simulink model "CHP_Test_Model"  (Simulink 8.1)
settings: Solver=ode4  StartTime=0.0  StopTime=40  FixedStep=Ts  MaxStep=1e-3  RelTol=1e-3
model workspace (MAT data in the model file):
  op_snapshot1 : opcond.OperatingPoint (value not decoded)
PostLoadFcn:
  | Ts=100e-6; HILLTOP_init;SIM_HIL=0; UnitTest_Breaker_init
InitFcn:
  | Ts=100e-6; HILLTOP_init;SIM_HIL=0; UnitTest_Breaker_init
undefined symbols (not defined in the file): fdesignblkfcn, gcbh, Left, NG_CHP, NG_CHP_lib, ph, relay_par, type, V
libraries: simulink x28, rtio_opalrt_common x21, rtlab x7, simulink_extras x6, artemis x5, powerlib x4, rteventslib x4, cables_lib x3, breaker_lib x3, rtio_generic_modbus x3, Load_lib x2, transformer_lib x2
(part 1 of 3)
settings Model: ARTEMISmethode_block_infos=$$__separator__$$CHP_Test_Model/ARTEMIS Guide$$__separator__$$  Creator=RE25624  LastModifiedBy=ed12083  BufferReuse=off
settings SolverCC: ZeroCrossAlgorithm=Adaptive
settings DataIOCC: ExternalInput=getinputstruct(op_snapshot1)  InitialState=getstatestruct(op_snapshot1)  LimitDataPoints=off  MaxDataPoints=90060  SignalLoggingSaveFormat=Dataset  SaveOutput=off  SignalLogging=off  DSMLogging=off  SaveTime=off  OutputSaveName=result
settings OptimizationCC: BlockReduction=off  OptimizeBlockIOStorage=off  BufferReuse=off  ExpressionFolding=off  LocalBlockOutputs=off
settings DebuggingCC: MaxConsecutiveZCsMsg=warning  IgnoredZcDiagnostic=none  SolverPrmCheckMsg=none  MultiTaskRateTransMsg=warning  FcnCallInpInsideContextMsg=EnableAllAsWarning  FrameProcessingCompatibilityMsg=error  ModelReferenceExtraNoncontSigs=warning  StrictBusMsg=None
settings ModelReferenceCC: UpdateModelReferenceTargets=IfOutOfDate
settings SFSimCC: SFSimEcho=off
settings GRTTargetCC: CodeReplacementLibrary=C89/C90 (ANSI)

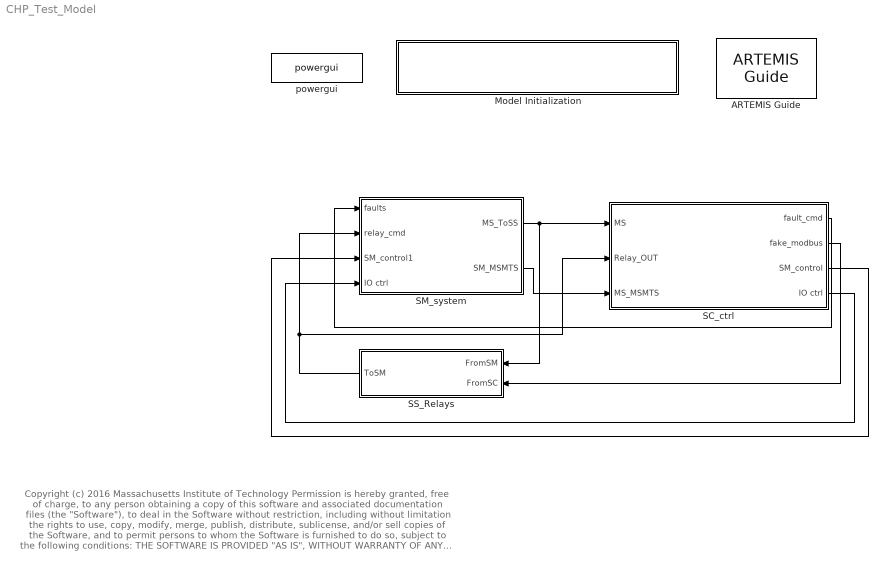
== system CHP_Test_Model ==
  note: Copyright (c) 2016 Massachusetts Institute of Technology
      | Permission is hereby granted, free of charge, to any person obtaining a copy of this software and associated documentation files (the "Software"), to deal
      | in the Software without restriction, including without limitation the rights to use, copy, modify, merge, publish, distribute, sublicense, and/or sell copies of the
      | Software, and to permit persons to whom the Software is furnished to do so, subject to the following conditions:
      |
      | THE SOFTWARE IS PROVIDED "AS IS", WITHOUT WARRANTY OF ANY KIND, EXPRESS OR IMPLIED, INCLUDING BUT NOT LIMITED TO THE
      | WARRANTIES OF MERCHANTABILITY, FITNESS FOR A PARTICULAR PURPOSE AND NONINFRINGEMENT. IN NO EVENT SHALL THE AUTHORS
      | OR COPYRIGHT HOLDERS BE LIABLE FOR ANY CLAIM, DAMAGES OR OTHER LIABILITY, WHETHER IN AN ACTION OF CONTRACT, TORT OR
      | OTHERWISE, ARISING FROM, OUT OF OR IN CONNECTION WITH THE SOFTWARE OR THE USE OR OTHER DEALINGS IN THE SOFTWARE.
  ARTEMIS Guide : artemis/ARTEMIS/ARTEMIS Guide  Tag=FTSSmethode_opal_4hx0r99  Description=5.0_z1  lock=on  Ts=Ts  opt=art5  dyna=off  nb_perm=4  RT_fullcomp=off  ssn=on  ssn_itvc=off  ssn_ivic=off  ssn_ext=off  ssn_solver=Art5 with Backward Euler nodal interface  ssn_impulse=off  ssn_quasimpulse=off  ssn_impulse_loop=2  paraExtinctionThy=off  Thy_Impulse=on  dtc=Off  dtc_opt=normal  ao=on  simtype=off  ct_mac=off  lin_mov=off  lsp=[0.001 2]  spike_skip=Disabled  dtc_extra=1  dtc_sws=normal  dtc_pied=0.5  SPSRulesBlock=SPSRules  tre=on  ctmm=off  LF=off  dpl_type=ARTEMiS DPL  rlc_type=off  custom_type=off  para=on  ssn_ImpulseLoopBlockedStateUpdate=2  ssn_mov_iter_number=5  ssn_switch_iter_number=5
  Model Initialization : Subsystem  AncestorBlock=artemis/Tools /Misc/Model Initialization  mask(Model Functions){InitFcnX=Ts=100e-6; HILLTOP_init;SIM_HIL=0; UnitTest_Breaker_init, prel=off, posl=on, inif=on, strf=off}
      mask prompts: InitFcnX "Initialisation"; prel "Preload Function"; posl "PostLoad Function"; inif "InitFcn"; strf "StartFcn"
      mask init:
      | currentBlock = gcb;
      | root = bdroot(currentBlock);
      | 
      | 
      | if ~strcmp(get_param(root,'BlockDiagramType'),'library')
      |     if prel==1
      |         set_param(root, 'PreLoadFcn', InitFcnX);
      |     else
      |         set_param(root, 'PreLoadFcn', '');
      |     end
      |     if inif==1
      |         set_param(root, 'InitFcn', InitFcnX);
      |     else
      |         set_param(root, 'InitFcn', '');
      |     end
      |     if strf==1
      |         set_param(root, 'StartFcn', InitFcnX);
      |     else
      |         set_param(root, 'StartFcn', '');
      |     end
      |     if posl==1
      |         set_param(root, 'PostLoadFcn', InitFcnX);
      |     else
      |         set_param(root, 'PostLoadFcn', '');
      |     end
      | end
      | 
      | pos = get_param(currentBlock, 'Position');
      | width = pos(3) - pos(1); height = pos(4) - pos(2);
      | txt = [ upper(root) '\n' '- InitFcn. . . . . '  get_param(root, 'InitFcn') ];
      settings: CopyFcn=set_param(gcb,'LinkStatus','inactive')
      mask Display: text(5, height*0.5, txt, 'horizontalAlignment', 'left', 'verticalAlignment', 'middle') ;
  SC_ctrl : Subsystem
  SM_system : Subsystem
  SS_Relays : Subsystem
  powergui : powerlib/powergui  Priority=2  SimulationMode=Discrete  SolverType=Tustin  SampleTime=Ts  frequency=60  SPID=off  DisableSnubberDevices=off  DisableRonSwitches=off  DisableVfSwitches=off  SwTol=0  Interpol=off  DisplayEquations=off  frequencyindice=0  Pbase=100e6  ErrMax=1e-4  Iterations=50  UnitsV=kV  UnitsW=MW  FunctionMessages=off  echomessages=off  HookPort=off  EnableUseOfTLC=off  x0status=blocks  RestoreLinks=warning  ResistiveCurrentMeasurement=off  Frange=logspace(0,3,50)  Ylog=off  Xlog=off  ShowGrid=off  save=off  variable=ZData  structure=0  ZoomFFT=on  StartTime=0.0  cycles=2  DisplayStyle=off  fundamental=60  FreqAxis=off  MaxFrequency=1000  frequencyindicesteady=1  RmsSteady=1  display=off  Ts=0  methode=off
  wires:
  SM_system/1(MS_ToSS) -> SC_ctrl/1(MS), SS_Relays/1(FromSM)
  SC_ctrl/1(fault_cmd) -> SM_system/1(faults)
  SS_Relays/1(ToSM) -> SM_system/2(relay_cmd), SC_ctrl/2(Relay_OUT)
  SC_ctrl/2(fake_modbus) -> SS_Relays/2(FromSC)
  SM_system/2(SM_MSMTS) -> SC_ctrl/3(MS_MSMTS)
  SC_ctrl/4(IO ctrl) -> SM_system/4(IO ctrl)
  SC_ctrl/3(SM_control) -> SM_system/3(SM_control1)

== system CHP_Test_Model/Model Initialization ==

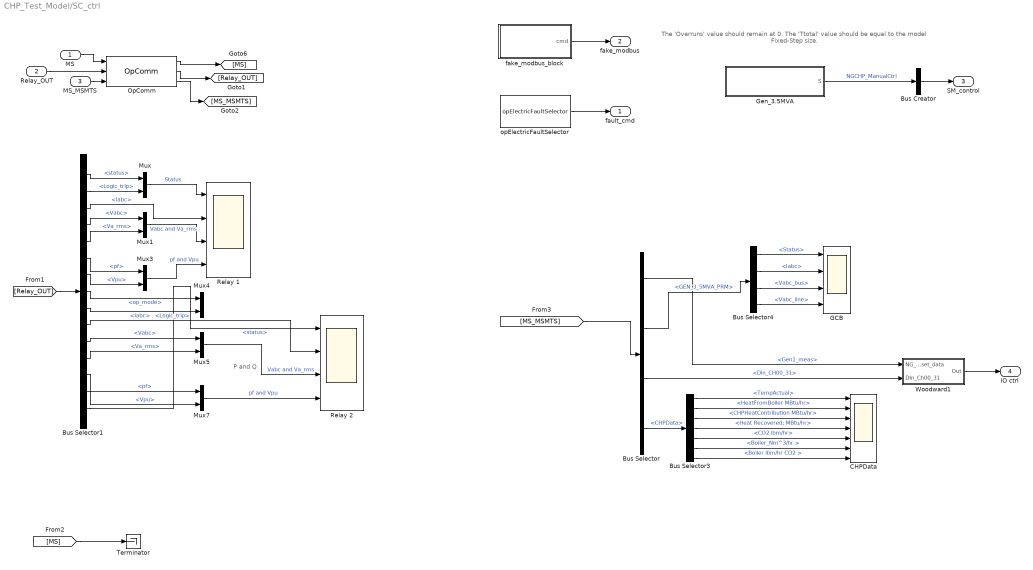
== system CHP_Test_Model/SC_ctrl ==
  note: P and Q
  note: The 'Overruns' value should remain at 0.
      | The 'Ttotal' value should be equal to the
      | model Fixed-Step size.
  MS : Inport
  Relay_OUT : Inport  Port=2
  MS_MSMTS : Inport  Port=3
  Bus Creator : BusCreator  Inputs=1
  Bus Selector : BusSelector  OutputSignals=Gen1_meas,GEN_3_5MVA_PRM,Din_CH00_31,CHPData
  Bus Selector1 : BusSelector  OutputSignals=relay_1.m.status,relay_1.Logic_trip,relay_1.m.Iabc,relay_1.m.Vabc,relay_1.m.Va_rms,relay_1.m.pf,relay_1.m.Vpu,relay_2.op_mode,relay_2.Logic_trip,relay_2.m.Iabc,relay_2.m.Vabc,relay_2.m.Va_rms,relay_2.m.pf,relay_2.m.Vpu,relay_2.m.status
  Bus Selector3 : BusSelector  OutputSignals=TempActual,HeatFromBoiler MBtu/hr,CHPHeatContribution MBtu/hr,Thermal data.Heat Recovered; MBtu/hr,Thermal data.CO2 lbm/hr,Boiler_Nm^3/hr ,Boiler lbm/hr CO2
  Bus Selector4 : BusSelector  OutputSignals=Status,Iabc,Vabc_bus,Vabc_line
  CHPData : Scope  NumInputPorts=7
      settings: ShowLegends=on  TimeRange=10  YMin=21.25~11~0~3.4058~2310.6~-5~-5  YMax=21.9~22~4~3.407~2311.5~5~5  SaveName=ScopeData5
  GCB : Scope  NumInputPorts=4
      settings: ShowLegends=on  TimeRange=0.02  YMin=0.95~-800~-100000~-100000  YMax=1.05~800~130000~130000
  Gen_3.5MVA : Subsystem
  Mux{,1,3..5,7} (6 alike) : Mux  Inputs=2
  OpComm : rtlab/OpComm  nbport=3  groupe_acq=1  subsys_rate=0  st=0  Synchronization=on  Interpolation=on  Threshold=1.0  Missed_Data=off  Sim_Time=off  Samples=off  dynSigOut=off  from_console=0  warning_done=off  writeOpCommFile=off  Offset=off
  Relay 1 : Scope  NumInputPorts=4
      settings: ShowLegends=on  TimeRange=1  YMin=1~-250~-15000~-1e+06  YMax=3~250~12500~2e+06  SaveName=ScopeData2
  Relay 2 : Scope  NumInputPorts=4
      settings: ShowLegends=on  TimeRange=1  YMin=0~-3000~-400~-100000  YMax=1~3000~400~1.4e+06  SaveName=ScopeData4
  Terminator : Terminator
  Woodward1 : Subsystem
  fake_modbus_block : Subsystem  mask(Fake Modbus Command){a=0, b=0, c=0, d=0, e=0, f=0}
      mask prompts: a "Relay#1: Reset"; b "Relay#1: Mode"; c "Relay#1: Group Settings"; d "Relay#2: Reset"; e "Relay#2: Mode"; f "Relay#2: Group Settings"
  opElectricFaultSelector : artemis/Tools /POW faults/opElectricFaultSelector  phase_a=on  phase_b=on  phase_c=on  gnd_fault=on  Tacq=1  Tst=[0.1 0 10]  enable_POW=off  angle_POW=[15 0 10]  Tdr="[0.5 0  10]"  fault_location_menu=No fault  T_init=2
  fault_cmd : Outport
  fake_modbus : Outport  Port=2
  SM_control : Outport  Port=3
  IO ctrl : Outport  Port=4
  wires:
  OpComm/1 -> [MS]
  MS/1 -> OpComm/1
  opElectricFaultSelector/1 -> fault_cmd/1
  [Relay_OUT] -> Bus Selector1/1
  OpComm/2 -> [Relay_OUT]
  Relay_OUT/1 -> OpComm/2
  Bus Selector1/3 -> Relay 1/2  "<Iabc>"
  Bus Selector1/1 -> Mux/1  "<status>"
  Bus Selector1/2 -> Mux/2  "<Logic_trip>"
  Bus Selector1/4 -> Mux1/1  "<Vabc>"
  Bus Selector1/5 -> Mux1/2  "<Va_rms>"
  Bus Selector1/6 -> Mux3/1  "<pf>"
  Bus Selector1/7 -> Mux3/2  "<Vpu>"
  Mux/1 -> Relay 1/1  "Status"
  Mux1/1 -> Relay 1/3  "Vabc and Va_rms"
  Mux3/1 -> Relay 1/4  "pf and Vpu"
  Bus Selector1/10 -> Relay 2/2  "<Iabc>"
  Bus Selector1/8 -> Mux4/1  "<op_mode>"
  Bus Selector1/9 -> Mux4/2  "<Logic_trip>"
  Bus Selector1/11 -> Mux5/1  "<Vabc>"
  Bus Selector1/12 -> Mux5/2  "<Va_rms>"
  Bus Selector1/13 -> Mux7/1  "<pf>"
  Bus Selector1/14 -> Mux7/2  "<Vpu>"
  Mux5/1 -> Relay 2/3  "Vabc and Va_rms"
  Mux7/1 -> Relay 2/4  "pf and Vpu"
  fake_modbus_block/1(cmd) -> fake_modbus/1
  Gen_3.5MVA/1(S) -> Bus Creator/1  "NGCHP_ManualCtrl"
  Bus Creator/1 -> SM_control/1
  Woodward1/1(Out) -> IO ctrl/1
  Bus Selector4/1 -> GCB/1  "<Status>"
  Bus Selector4/2 -> GCB/2  "<Iabc>"
  Bus Selector4/3 -> GCB/3  "<Vabc_bus>"
  Bus Selector4/4 -> GCB/4  "<Vabc_line>"
  Bus Selector/2 -> Bus Selector4/1  "<GEN_3_5MVA_PRM>"
  Bus Selector/1 -> Woodward1/1(NG_genset_data)  "<Gen1_meas>"
  Bus Selector/3 -> Woodward1/2(DIn_Ch00_31)  "<Din_CH00_31>"
  MS_MSMTS/1 -> OpComm/3
  [MS_MSMTS] -> Bus Selector/1
  OpComm/3 -> [MS_MSMTS]
  Bus Selector/4 -> Bus Selector3/1  "<CHPData>"
  Bus Selector3/1 -> CHPData/1  "<TempActual>"
  Bus Selector3/5 -> CHPData/5  "<CO2 lbm/hr>"
  Bus Selector3/2 -> CHPData/2  "<HeatFromBoiler MBtu/hr>"
  Bus Selector3/3 -> CHPData/3  "<CHPHeatContribution MBtu/hr>"
  Bus Selector3/4 -> CHPData/4  "<Heat Recovered; MBtu/hr>"
  Bus Selector1/15 -> Relay 2/1  "<status>"
  [MS] -> Terminator/1
  Bus Selector3/6 -> CHPData/6  "<Boiler_Nm^3/hr >"
  Bus Selector3/7 -> CHPData/7  "<Boiler lbm/hr CO2 >"

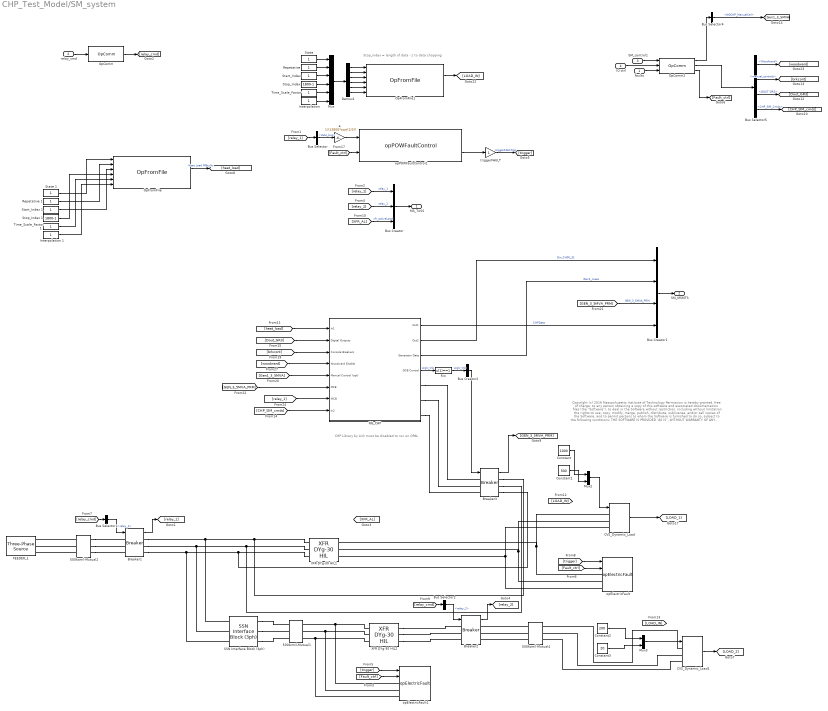
== system CHP_Test_Model/SM_system ==
  note: CHP Library by Link must be disabled
      | to run on OPAL
  note: Stop_index = length of data - 1 to data chopping
  note: Copyright (c) 2016 Massachusetts Institute of Technology
      | Permission is hereby granted, free of charge, to any person obtaining a copy of this software and associated documentation files (the "Software"), to deal
      | in the Software without restriction, including without limitation the rights to use, copy, modify, merge, publish, distribute, sublicense, and/or sell copies of the
      | Software, and to permit persons to whom the Software is furnished to do so, subject to the following conditions:
      |
      | THE SOFTWARE IS PROVIDED "AS IS", WITHOUT WARRANTY OF ANY KIND, EXPRESS OR IMPLIED, INCLUDING BUT NOT LIMITED TO THE
      | WARRANTIES OF MERCHANTABILITY, FITNESS FOR A PARTICULAR PURPOSE AND NONINFRINGEMENT. IN NO EVENT SHALL THE AUTHORS
      | OR COPYRIGHT HOLDERS BE LIABLE FOR ANY CLAIM, DAMAGES OR OTHER LIABILITY, WHETHER IN AN ACTION OF CONTRACT, TORT OR
      | OTHERWISE, ARISING FROM, OUT OF OR IN CONNECTION WITH THE SOFTWARE OR THE USE OR OTHER DEALINGS IN THE SOFTWARE
  faults : Inport
  relay_cmd : Inport  Port=2
  SM_control1 : Inport  Port=3
  IO ctrl : Inport  Port=4
  500kcmil-Mutual1 : cables_lib/500kcmil-Mutual  length=5000  par_sets=1  ratio=3
  500kcmil-Mutual2 : cables_lib/500kcmil-Mutual  length=5000  par_sets=1  ratio=3
  500kcmil-Mutual4 : cables_lib/500kcmil-Mutual  length=1100  par_sets=1  ratio=3
  Breaker1 : breaker_lib/Breaker  Ts=Ts  mech_delay=cb_mech_delay
  Breaker2 : breaker_lib/Breaker  Ts=Ts  mech_delay=cb_mech_delay
  Breaker3 : breaker_lib/Breaker  Ts=Ts  mech_delay=cb_mech_delay
  Bus Creator : BusCreator  Inputs=3
  Bus Creator1 : BusCreator
  Bus Creator2 : BusCreator  Inputs=1
  Bus Selector : BusSelector  OutputSignals=Vabc_bus
  Bus Selector1 : BusSelector  OutputSignals=relay_1
  Bus Selector2 : BusSelector  OutputSignals=relay_2
  Bus Selector4 : BusSelector  OutputSignals=NGCHP_ManualCtrl
  Bus Selector5 : BusSelector  OutputSignals=Woodward,manual_controls,DOUT GR3,DOUT GR3.16 DOUT GR3.CHP_SIM_Cmds
  CVS_Dynamic_Load : Load_lib/CVS_Dynamic_Load  V=480  Ts=Ts
  CVS_Dynamic_Load1 : Load_lib/CVS_Dynamic_Load  V=460  Ts=Ts
  Constant : Constant  Value=1000
  Constant1 : Constant  Value=500
  Constant2 : Constant  Value=200
  Constant3 : Constant  Value=20
  Demux1 : Demux  Outputs=6
  FEEDER_1 : powerlib/Electrical Sources/Three-Phase Source  Voltage=13800  PhaseAngle=0  Frequency=60  InternalConnection=Yg  SpecifyImpedance=on  Resistance=0.8929  Inductance=16.58e-3  ShortCircuitLevel=375e6  BaseVoltage=13800  XRratio=7.9  BusType=swing  Pref=0  Qref=0  Qmin=-inf  Qmax=inf
  Fcn : Fcn  Expr=u(1)==1
  "Interpolation " : Constant
  Interpolation 1 : Constant
  Mux : Mux  Inputs=6
  Mux2 : Mux  Inputs=2
  Mux3 : Mux  Inputs=2
  NG_CHP : Subsystem  AncestorBlock=NG_CHP_lib/NG_CHP
  OpComm : rtlab/OpComm  nbport=1  groupe_acq=1  subsys_rate=0  st=0  Synchronization=on  Interpolation=on  Threshold=1.0  Missed_Data=off  Sim_Time=off  Samples=off  dynSigOut=off  from_console=0  warning_done=off  writeOpCommFile=off  Offset=off
  OpComm2 : rtlab/OpComm  nbport=3  groupe_acq=1  subsys_rate=0  st=0  Synchronization=on  Interpolation=on  Threshold=1.0  Missed_Data=off  Sim_Time=off  Samples=off  dynSigOut=off  from_console=1  warning_done=off  writeOpCommFile=off  Offset=off
  OpFromFile : rtlab/DataLogging/OpFromFile  filename_mode=Static (same filename all the time)  reload_mode=Next time model is paused (Real-Time)  init_file_id=0  filename=HeatLoad.mat  rtpath='./'  nrtpath='.\'  sample_time=Ts
  OpFromFile1 : rtlab/DataLogging/OpFromFile  filename_mode=Static (same filename all the time)  reload_mode=Next time model is paused (Real-Time)  init_file_id=0  filename=one_min_data.mat  rtpath='./'  nrtpath='.\'  sample_time=0
  "Repetative " : Constant
  Repetative 1 : Constant
  SSN Interface Block (3ph) : ssn_lib/SSN Interface Block (3ph)  nb_phase=3  nb_port=2  p1_type=V-type(Left)  p2_type=V-type (Right)  p3_type=V-type(Left)  p4_type=V-type(Left)  p5_type=V-type(Left)  p6_type=V-type(Left)  p7_type=V-type(Left)  p8_type=V-type(Left)  p9_type=V-type(Left)  p10_type=V-type(Left)  p11_type=V-type(Left)  p12_type=V-type(Left)  p13_type=V-type(Left)  p14_type=V-type(Left)  p15_type=V-type(Left)  p16_type=V-type(Left)  I_port_shunt_resistance=1e9
  "Start_Index " : Constant
  Start_Index 1 : Constant
  "State " : Constant
  State 1 : Constant
  "Stop_Index " : Constant  Value=1800-1
  Stop_Index 1 : Constant  Value=1800-1
  "Time_Scale_Factor " : Constant
  Time_Scale_Factor 1 : Constant
  XFR DYg-30 HIL1 : transformer_lib/XFR DYg-30 HIL  Rating=2500  Vp=13800  Vs=480  Z=5.18  XR=2.5
  XFR DYg-30 HIL2 : transformer_lib/XFR DYg-30 HIL  Rating=2500  Vp=13800  Vs=460  Z=5.18  XR=2.5
  a : Gain  Gain=1/(13800*sqrt(2/3))
  opElectricFault : artemis/Tools /POW faults/opElectricFault  FaultLocation=location 2  FaultResistance=0.0001  GroundResistance=0.0001  InitialStates=[0 0 0]  SnubberResistance=1e6  SnubberCapacitance=inf
  opElectricFault1 : artemis/Tools /POW faults/opElectricFault  FaultLocation=location 1  FaultResistance=0.0001  GroundResistance=0.0001  InitialStates=[0 0 0]  SnubberResistance=1e6  SnubberCapacitance=inf
  opPOWFaultControl1 : artemis/Tools /POW faults/opPOWFaultControl  Ts=Ts  usePLL=off  Fgrid=60  PLL_k=[180 3200 1]  vol_sel=1: rising zero-corssing  SyncPhase_menu=A  T_acq=0.8
  triggerFAULT : Gain
  MS_ToSS : Outport
  SM_MSMTS : Outport  Port=2
  wires:
  Breaker1/1 -> [relay_1]
  [Fault_ctrl] -> opPOWFaultControl1/2
  opPOWFaultControl1/2 -> triggerFAULT/1
  triggerFAULT/1 -> [trigger]  "triggerFAULTsig"
  [Fault_ctrl] -> opElectricFault/2
  [trigger] -> opElectricFault/1
  [relay_1] -> Bus Selector/1
  Bus Selector/1 -> a/1  "<Vabc_bus>"
  a/1 -> opPOWFaultControl1/1
  Breaker2/1 -> [relay_2]
  [Fault_ctrl] -> opElectricFault1/2
  [trigger] -> opElectricFault1/1
  [relay_1] -> Bus Creator/1  "relay_1"
  [relay_2] -> Bus Creator/2  "relay_2"
  Bus Creator/1 -> MS_ToSS/1
  [relay_cmd] -> Bus Selector1/1
  Bus Selector1/1 -> Breaker1/1  "<relay_1>"
  [relay_cmd] -> Bus Selector2/1
  Bus Selector2/1 -> Breaker2/1  "<relay_2>"
  OpComm/1 -> [relay_cmd]
  OpComm2/3 -> [Fault_ctrl]
  faults/1 -> OpComm2/3
  relay_cmd/1 -> OpComm/1
  [XFR_AL] -> Bus Creator/3  "xfr_activeLoad"
  Breaker3/1 -> [GEN_3_5MVA_PRM]
  SM_control1/1 -> OpComm2/1
  OpComm2/1 -> Bus Selector4/1
  Bus Selector4/1 -> [Gen1_3_5MVA]  "<NGCHP_ManualCtrl>"
  OpComm2/2 -> Bus Selector5/1
  Bus Selector5/1 -> [woodward]  "<Woodward>"
  IO ctrl/1 -> OpComm2/2
  Bus Selector5/3 -> [Dout_GR3]  "<DOUT GR3>"
  Bus Selector5/2 -> [brkcont]  "<manual_controls>"
  [GEN_3_5MVA_PRM] -> Bus Creator1/3  "GEN_3_5MVA_PRM"
  Bus Creator1/1 -> SM_MSMTS/1
  NG_CHP/3(Generator Data) -> Bus Creator1/2  "Gen1_meas"
  NG_CHP/2(Out2) -> Bus Creator1/1  "Din_CH00_31"
  ? -> [XFR_AL]
  State 1/1 -> OpFromFile/1
  Interpolation 1/1 -> OpFromFile/6
  Time_Scale_Factor 1/1 -> OpFromFile/5
  Stop_Index 1/1 -> OpFromFile/4
  Start_Index 1/1 -> OpFromFile/3
  Repetative 1/1 -> OpFromFile/2
  "Stop_Index "/1 -> Mux/4
  Demux1/2 -> OpFromFile1/2
  Demux1/5 -> OpFromFile1/5
  OpFromFile1/2 -> [LOAD_IN]
  "Interpolation "/1 -> Mux/6
  Mux/1 -> Demux1/1
  Demux1/4 -> OpFromFile1/4
  Demux1/1 -> OpFromFile1/1
  Demux1/6 -> OpFromFile1/6
  Demux1/3 -> OpFromFile1/3
  "Start_Index "/1 -> Mux/3
  "Time_Scale_Factor "/1 -> Mux/5
  "Repetative "/1 -> Mux/2
  "State "/1 -> Mux/1
  CVS_Dynamic_Load/1 -> [LOAD_1]
  CVS_Dynamic_Load1/1 -> [LOAD_2]
  Constant1/1 -> Mux2/2
  Constant/1 -> Mux2/1
  Constant2/1 -> Mux3/1
  Constant3/1 -> Mux3/2
  [Dout_GR3] -> NG_CHP/2(Digital Outputs)
  [brkcont] -> NG_CHP/3(Console Breakers)
  [woodward] -> NG_CHP/4(Woodward Enable)
  [Gen1_3_5MVA] -> NG_CHP/5(Manual Control (opt))
  [GEN_3_5MVA_PRM] -> NG_CHP/6(GCB)
  [relay_1] -> NG_CHP/7(MCB)
  NG_CHP/1(Out1) -> Bus Creator1/4  "CHPData"
  Bus Creator2/1 -> Breaker3/1
  Bus Selector5/4 -> [CHP_SIM_cmds]  "<CHP_SIM_Cmds>"
  OpFromFile/2 -> [heat_load]  "Heat Load MBtu/hr"
  [heat_load] -> NG_CHP/1(In1)
  [CHP_SIM_cmds] -> NG_CHP/8(In2)
  NG_CHP/4(GCB Control) -> Fcn/1  "Logic_trip"
  Fcn/1 -> Bus Creator2/1  "Logic_trip"
  Mux2/1 -> CVS_Dynamic_Load/1
  Mux3/1 -> CVS_Dynamic_Load1/1
  connections:
  500kcmil-Mutual2/LConn2 -- FEEDER_1/RConn2
  500kcmil-Mutual2/LConn1 -- FEEDER_1/RConn1
  500kcmil-Mutual2/LConn3 -- FEEDER_1/RConn3
  XFR DYg-30 HIL2/LConn1 -- opElectricFault1/LConn1 -- 500kcmil-Mutual1/RConn1
  XFR DYg-30 HIL2/LConn2 -- opElectricFault1/LConn2 -- 500kcmil-Mutual1/RConn2
  XFR DYg-30 HIL2/LConn3 -- opElectricFault1/LConn3 -- 500kcmil-Mutual1/RConn3
  500kcmil-Mutual2/RConn1 -- Breaker1/LConn1
  500kcmil-Mutual2/RConn2 -- Breaker1/LConn2
  500kcmil-Mutual2/RConn3 -- Breaker1/LConn3
  Breaker1/RConn1 -- SSN Interface Block (3ph)/LConn1 -- Breaker3/RConn1 -- XFR DYg-30 HIL1/LConn1
  Breaker1/RConn2 -- SSN Interface Block (3ph)/LConn2 -- Breaker3/RConn2 -- XFR DYg-30 HIL1/LConn2
  Breaker1/RConn3 -- SSN Interface Block (3ph)/LConn3 -- Breaker3/RConn3 -- XFR DYg-30 HIL1/LConn3
  opElectricFault/LConn2 -- CVS_Dynamic_Load/LConn2 -- XFR DYg-30 HIL1/RConn2
  opElectricFault/LConn1 -- CVS_Dynamic_Load/LConn1 -- XFR DYg-30 HIL1/RConn1
  opElectricFault/LConn3 -- CVS_Dynamic_Load/LConn3 -- XFR DYg-30 HIL1/RConn3
  SSN Interface Block (3ph)/RConn2 -- 500kcmil-Mutual1/LConn2
  SSN Interface Block (3ph)/RConn1 -- 500kcmil-Mutual1/LConn1
  SSN Interface Block (3ph)/RConn3 -- 500kcmil-Mutual1/LConn3
  XFR DYg-30 HIL2/RConn3 -- Breaker2/LConn3
  XFR DYg-30 HIL2/RConn2 -- Breaker2/LConn2
  XFR DYg-30 HIL2/RConn1 -- Breaker2/LConn1
  500kcmil-Mutual4/LConn1 -- Breaker2/RConn1
  500kcmil-Mutual4/LConn2 -- Breaker2/RConn2
  500kcmil-Mutual4/LConn3 -- Breaker2/RConn3
  NG_CHP/RConn1 -- Breaker3/LConn1
  NG_CHP/RConn2 -- Breaker3/LConn2
  NG_CHP/RConn3 -- Breaker3/LConn3
  CVS_Dynamic_Load1/LConn3 -- 500kcmil-Mutual4/RConn3
  CVS_Dynamic_Load1/LConn2 -- 500kcmil-Mutual4/RConn2
  CVS_Dynamic_Load1/LConn1 -- 500kcmil-Mutual4/RConn1

== system CHP_Test_Model/SS_Relays ==
  FromSM : Inport
  FromSC : Inport  Port=2
  Bus Creator : BusCreator  Inputs=2
  Bus Selector : BusSelector  OutputSignals=relay_1,relay_2
  Bus Selector1 : BusSelector  OutputSignals=Relay_1,Relay_2
  Generic_Relay_v2_1 : relay_modbus_lib/Generic_Relay_v2_1  Ts=Ts  relay_settings=[relay_par(1,:)]
  Generic_Relay_v2_2 : relay_modbus_lib/Generic_Relay_v2_1  Ts=Ts  relay_settings=[relay_par(2,:)]
  Modbus device : rtio_generic_modbus/Modbus device  conf_name=F1_relay_cfg1.opal  conf_name_mask=F1_relay_cfg1.xls  sample_time=Ts
  Modbus device1 : rtio_generic_modbus/Modbus device  conf_name=F1_relay_cfg2.opal  conf_name_mask=F1_relay_cfg2.xls  sample_time=Ts
  OpComm : rtlab/OpComm  nbport=1  groupe_acq=1  subsys_rate=0  st=0  Synchronization=on  Interpolation=on  Threshold=1.0  Missed_Data=off  Sim_Time=off  Samples=off  dynSigOut=off  from_console=0  warning_done=off  writeOpCommFile=off  Offset=off
  OpComm1 : rtlab/OpComm  nbport=1  groupe_acq=1  subsys_rate=0  st=0  Synchronization=on  Interpolation=on  Threshold=1.0  Missed_Data=off  Sim_Time=off  Samples=off  dynSigOut=off  from_console=1  warning_done=off  writeOpCommFile=off  Offset=off
  ToSM : Outport
  wires:
  OpComm/1 -> Bus Selector/1
  FromSM/1 -> OpComm/1
  Bus Selector/1 -> Generic_Relay_v2_1/1  "<relay_1>"
  Bus Selector/2 -> Generic_Relay_v2_2/1  "<relay_2>"
  Generic_Relay_v2_1/1 -> Bus Creator/1  "relay_1"
  Generic_Relay_v2_2/1 -> Bus Creator/2  "relay_2"
  Bus Creator/1 -> ToSM/1
  FromSC/1 -> OpComm1/1
  OpComm1/1 -> Bus Selector1/1
  Bus Selector1/2 -> Generic_Relay_v2_2/2  "<Relay_2>"
  Bus Selector1/1 -> Generic_Relay_v2_1/2  "<Relay_1>"
  Generic_Relay_v2_1/2 -> Modbus device/1
  Generic_Relay_v2_2/2 -> Modbus device1/1

== system CHP_Test_Model/SC_ctrl/Gen_3.5MVA ==
  1 - PQ 2 - PV 3 - VF : Constant  Value=3
  2.5 - 130 s : DiscretePulseGenerator  Period=150/Ts  PulseWidth=127.5/Ts  PhaseDelay=2.5/Ts  SampleTime=Ts
  Bus Creator : BusCreator  Inputs=6
  DONOTCHANGE : Constant
  Enable = 1 Disable = 0 : Constant  Value=0
  F : simulink/Math Operations/Slider Gain  low=0.97  gain=1  high=1.03
  Fcmd pu : Constant  Value=1.0
  P : simulink/Math Operations/Slider Gain  low=0  gain=0.8  high=1.1
  Pfactor : Gain  Gain=.9
  Q : simulink/Math Operations/Slider Gain  low=0.01  gain=0.2  high=0.4
  Qfactor : Gain  Gain=.43
  S Profile : simulink/Sources/Repeating Sequence Stair  OutValues=[.1 .1 .1 .1 .1 .1 .5 .5 .5 .5 .5 .5 .5 .5 .5 .5 .5 .5 1 1 1 1 1 ]  tsamp=[5 Ts]  OutMin=[]  OutMax=[]  OutDataTypeStr=Inherit: Inherit via back propagation  OutDataType=fixdt(0,8)  ConRadixGroup=Best Precision: Vector-wise  OutScaling=2^-12
  V : simulink/Math Operations/Slider Gain  low=0.9  gain=1  high=1.1
  VF - to end : simulink/Sources/Repeating Sequence Stair  OutValues=[3 3 3 3 3 3 3 3 3 3 3 3 3 3 3 3 3 3 3 3 3 3 3 3 3 3 3 3 3 3 3 ]  tsamp=[5 Ts]  OutMin=[]  OutMax=[]  OutDataTypeStr=Inherit: Inherit via back propagation  OutDataType=fixdt(0,8)  ConRadixGroup=Best Precision: Vector-wise  OutScaling=2^-12
  Vcmd pu : Constant
  S : Outport
  wires:
  Pfactor/1 -> Bus Creator/1  "P"
  Fcmd pu/1 -> Bus Creator/4  "F"
  2.5 - 130 s/1 -> Bus Creator/6  "Enable"
  VF - to end/1 -> Bus Creator/5  "Mode"
  Vcmd pu/1 -> Bus Creator/3  "V"
  Qfactor/1 -> Bus Creator/2  "Q"
  S Profile/1 -> Pfactor/1, Qfactor/1  "P"
  Bus Creator/1 -> S/1
  DONOTCHANGE/1 -> F/1, V/1, Q/1, P/1

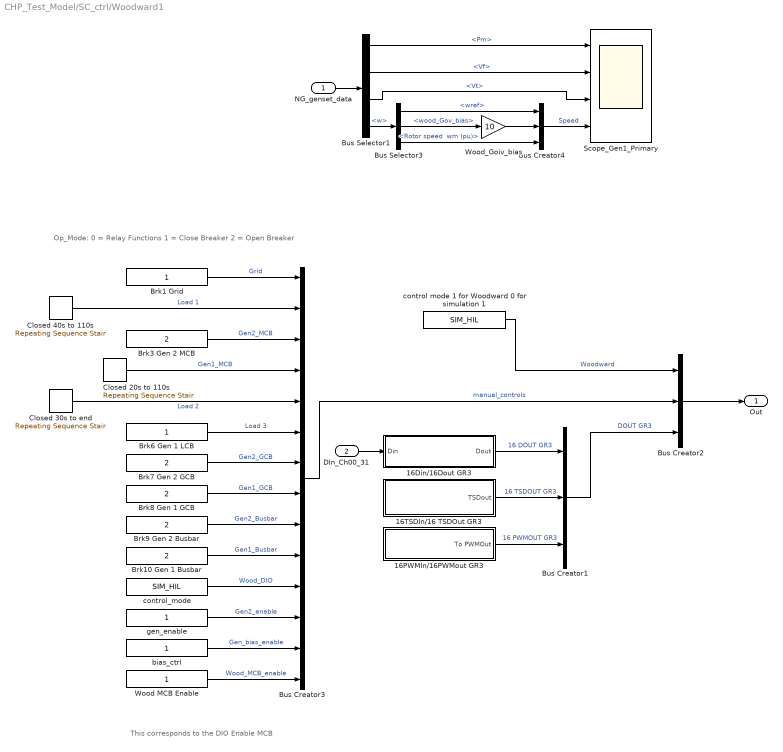
== system CHP_Test_Model/SC_ctrl/Woodward1 ==
  note: This corresponds to
      | the DIO Enable MCB
  note: Op_Mode:
      | 0 = Relay Functions
      | 1 = Close Breaker
      | 2 = Open Breaker
  NG_genset_data : Inport
  DIn_Ch00_31 : Inport  Port=2
  16Din/16Dout GR3 : Subsystem
  16PWMIn/16PWMout GR3 : Subsystem
  16TSDIn/16 TSDOut GR3 : Subsystem
  Brk1 Grid : Constant
  Brk10 Gen 1 Busbar : Constant  Value=2
  Brk3 Gen 2 MCB : Constant  Value=2
  Brk6 Gen 1 LCB : Constant
  Brk7 Gen 2 GCB : Constant  Value=2
  Brk8 Gen 1 GCB : Constant  Value=2
  Brk9 Gen 2 Busbar : Constant  Value=2
  Bus Creator1 : BusCreator  Inputs=3
  Bus Creator2 : BusCreator  Inputs=3
  Bus Creator3 : BusCreator  Inputs=14
  Bus Creator4 : BusCreator  Inputs=3
  Bus Selector1 : BusSelector  OutputSignals=Pm,Vf,Vt,w
  Bus Selector3 : BusSelector  OutputSignals="wref,w.wood_Gov_bias,w.Rotor speed  wm (pu)"
  Closed 20s to 110s : simulink/Sources/Repeating Sequence Stair  OutValues=[2 2 2 2 1 1 1 1 1 1 1 1 1 1 1 1 1 1 1 1 1 1 2 2 2 2 2]  tsamp=[5 Ts]  OutMin=[]  OutMax=[]  OutDataTypeStr=double  OutputDataTypeScalingMode=double  OutDataType=fixdt(0,8)  ConRadixGroup=Best Precision: Vector-wise  OutScaling=2^-12
  Closed 30s to end : simulink/Sources/Repeating Sequence Stair  OutValues=[2 2 2 2 2 2 1 1 1 1 1 1 1 1 1 1 1 1 1 1 1 1 ]  tsamp=[5 Ts]  OutMin=[]  OutMax=[]  OutDataTypeStr=double  OutputDataTypeScalingMode=double  OutDataType=fixdt(0,8)  ConRadixGroup=Best Precision: Vector-wise  OutScaling=2^-12
  Closed 40s to 110s : simulink/Sources/Repeating Sequence Stair  OutValues=[2 2 2 2 2 2 2 2 1 1 1 1 1 1 1 1 1 1 1 1 1 1 2 2 2]  tsamp=[5 Ts]  OutMin=[]  OutMax=[]  OutDataTypeStr=double  OutputDataTypeScalingMode=double  OutDataType=fixdt(0,8)  ConRadixGroup=Best Precision: Vector-wise  OutScaling=2^-12
  Scope_Gen1_Primary : Scope  NumInputPorts=4
      settings: ShowLegends=on  TimeRange=10  YMin=-0.05~-0.5~0~0  YMax=0.75~5.5~1.1~1.1  SaveName=ScopeData4
  Wood MCB Enable : Constant
  Wood_Goiv_bias : Gain  Gain=10
  bias_ctrl : Constant
  control mode 1 for Woodward 0 for simulation 1 : Constant  Value=SIM_HIL
  control_mode : Constant  Value=SIM_HIL
  gen_enable : Constant
  Out : Outport
  wires:
  Brk1 Grid/1 -> Bus Creator3/1  "Grid"
  Brk10 Gen 1 Busbar/1 -> Bus Creator3/10  "Gen1_Busbar"
  Brk9 Gen 2 Busbar/1 -> Bus Creator3/9  "Gen2_Busbar"
  Wood_Goiv_bias/1 -> Bus Creator4/2
  Brk8 Gen 1 GCB/1 -> Bus Creator3/8  "Gen1_GCB"
  Brk7 Gen 2 GCB/1 -> Bus Creator3/7  "Gen2_GCB"
  Brk6 Gen 1 LCB/1 -> Bus Creator3/6  "Load 3"
  Closed 30s to end/1 -> Bus Creator3/5  "Load 2"
  Bus Creator4/1 -> Scope_Gen1_Primary/4  "Speed"
  Bus Selector3/3 -> Bus Creator4/3  "<Rotor speed  wm (pu)>"
  Bus Selector3/2 -> Wood_Goiv_bias/1  "<wood_Gov_bias>"
  Bus Selector3/1 -> Bus Creator4/1  "<wref>"
  Bus Selector1/4 -> Bus Selector3/1  "<w>"
  Wood MCB Enable/1 -> Bus Creator3/14  "Wood_MCB_enable"
  NG_genset_data/1 -> Bus Selector1/1
  Bus Selector1/3 -> Scope_Gen1_Primary/3  "<Vt>"
  Bus Selector1/2 -> Scope_Gen1_Primary/2  "<Vf>"
  Bus Selector1/1 -> Scope_Gen1_Primary/1  "<Pm>"
  DIn_Ch00_31/1 -> 16Din/16Dout GR3/1(Din)
  Bus Creator2/1 -> Out/1
  bias_ctrl/1 -> Bus Creator3/13  "Gen_bias_enable"
  gen_enable/1 -> Bus Creator3/12  "Gen2_enable"
  control_mode/1 -> Bus Creator3/11  "Wood_DIO"
  Closed 20s to 110s/1 -> Bus Creator3/4  "Gen1_MCB"
  Brk3 Gen 2 MCB/1 -> Bus Creator3/3  "Gen2_MCB"
  Closed 40s to 110s/1 -> Bus Creator3/2  "Load 1"
  Bus Creator3/1 -> Bus Creator2/2  "manual_controls"
  Bus Creator1/1 -> Bus Creator2/3  "DOUT GR3"
  16PWMIn/16PWMout GR3/1(To PWMOut) -> Bus Creator1/3  "16 PWMOUT GR3"
  16TSDIn/16 TSDOut GR3/1(TSDout) -> Bus Creator1/2  "16 TSDOUT GR3"
  16Din/16Dout GR3/1(Dout) -> Bus Creator1/1  "16 DOUT GR3"
  control mode 1 for Woodward 0 for simulation 1/1 -> Bus Creator2/1  "Woodward"

== system CHP_Test_Model/SC_ctrl/fake_modbus_block ==
  Bus Creator : BusCreator  Inputs=2
  Constant : Constant  Value=a
  Constant1 : Constant  Value=c
  Constant2 : Constant  Value=b
  Constant3 : Constant  Value=d
  Constant4 : Constant  Value=f
  Constant5 : Constant  Value=e
  Mux11 : Mux  Inputs=3
  Mux12 : Mux  Inputs=3
  cmd : Outport
  wires:
  Bus Creator/1 -> cmd/1
  Mux11/1 -> Bus Creator/1  "Relay_1"
  Constant5/1 -> Mux12/2  "mode"
  Constant4/1 -> Mux12/3  "setting_grp"
  Constant3/1 -> Mux12/1  "reset"
  Mux12/1 -> Bus Creator/2  "Relay_2"
  Constant1/1 -> Mux11/3  "setting_grp"
  Constant2/1 -> Mux11/2  "mode"
  Constant/1 -> Mux11/1  "reset"

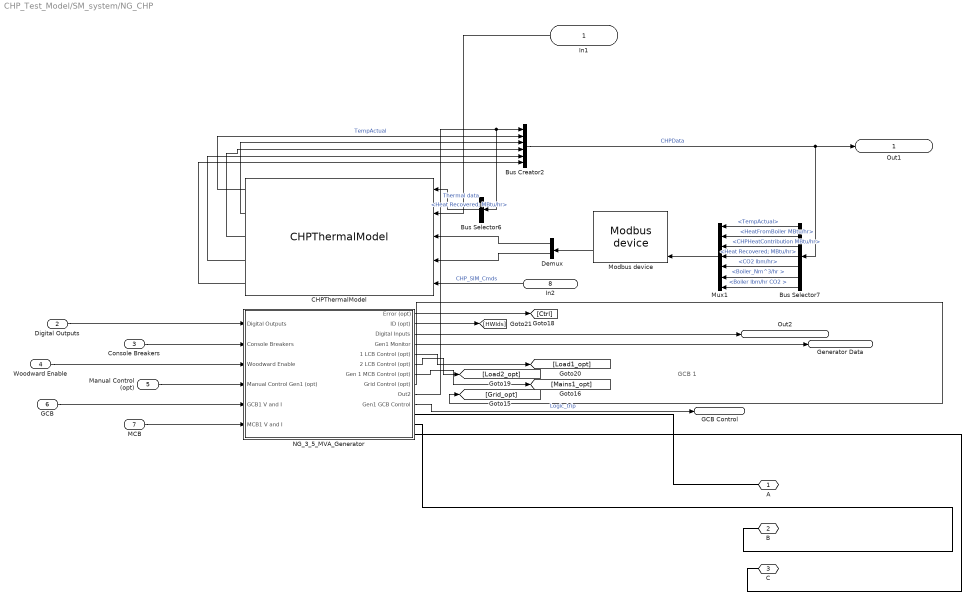
== system CHP_Test_Model/SM_system/NG_CHP ==
  note: GCB 1
  In1 : Inport
  Digital Outputs : Inport  Port=2
  Console Breakers : Inport  Port=3
  Woodward Enable : Inport  Port=4
  Manual Control (opt) : Inport  Port=5
  GCB : Inport  Port=6
  MCB : Inport  Port=7
  In2 : Inport  Port=8
  Bus Creator2 : BusCreator  Inputs=6
  Bus Selector6 : BusSelector  OutputSignals=Heat Recovered; MBtu/hr
  Bus Selector7 : BusSelector  OutputSignals=TempActual,HeatFromBoiler MBtu/hr,CHPHeatContribution MBtu/hr,Thermal data.Heat Recovered; MBtu/hr,Thermal data.CO2 lbm/hr,Boiler_Nm^3/hr ,Boiler lbm/hr CO2
  CHPThermalModel : CHP_Model_lib/CHPThermalModel  SIM_HIL=SIM_HIL
  Demux : Demux  Outputs=2
  Modbus device : rtio_generic_modbus/Modbus device  conf_name=CHP_slave_cfg.opal  conf_name_mask=CHP_slave_cfg.xls  sample_time=Ts
  Mux1 : Mux  Inputs=7
  NG_3_5_MVA_Generator : Subsystem
  A : PMIOPort  Tag=A  Port=1  Side=Right
      settings: AttributesFormatString=A
  B : PMIOPort  Port=2  Side=Right
  C : PMIOPort  Port=3  Side=Right
  Out1 : Outport
  Out2 : Outport  Port=2
  Generator Data : Outport  Port=3
  GCB Control : Outport  Port=4
  wires:
  Bus Selector7/3 -> Mux1/3  "<CHPHeatContribution MBtu/hr>"
  CHPThermalModel/1 -> Bus Creator2/2  "TempActual"
  Demux/2 -> CHPThermalModel/4
  CHPThermalModel/2 -> Bus Creator2/3
  NG_3_5_MVA_Generator/7(Gen 1 MCB Control (opt)) -> [Mains1_opt]
  Console Breakers/1 -> NG_3_5_MVA_Generator/2(Console Breakers)
  NG_3_5_MVA_Generator/8(Grid Control (opt)) -> [Grid_opt]
  Digital Outputs/1 -> NG_3_5_MVA_Generator/1(Digital Outputs)
  Bus Selector7/2 -> Mux1/2  "<HeatFromBoiler MBtu/hr>"
  Bus Selector7/5 -> Mux1/5  "<CO2 lbm/hr>"
  Bus Selector7/4 -> Mux1/4  "<Heat Recovered; MBtu/hr>"
  Bus Selector7/1 -> Mux1/1  "<TempActual>"
  In1/1 -> CHPThermalModel/2
  Mux1/1 -> Modbus device/4
  Demux/1 -> CHPThermalModel/3
  CHPThermalModel/3 -> Bus Creator2/4
  NG_3_5_MVA_Generator/9(Out2) -> Bus Selector6/1, Bus Creator2/1  "Thermal data"
  Modbus device/2 -> Demux/1
  NG_3_5_MVA_Generator/2(ID (opt)) -> [HWIds]
  Woodward Enable/1 -> NG_3_5_MVA_Generator/3(Woodward Enable)
  NG_3_5_MVA_Generator/1(Error (opt)) -> [Ctrl]
  NG_3_5_MVA_Generator/4(Gen1 Monitor) -> Generator Data/1
  GCB/1 -> NG_3_5_MVA_Generator/5(GCB1 V and I)
  Manual Control (opt)/1 -> NG_3_5_MVA_Generator/4(Manual Control Gen1 (opt))
  NG_3_5_MVA_Generator/6(2 LCB Control (opt)) -> [Load2_opt]
  MCB/1 -> NG_3_5_MVA_Generator/6(MCB1 V and I)
  NG_3_5_MVA_Generator/5(1 LCB Control (opt)) -> [Load1_opt]
  Bus Selector6/1 -> CHPThermalModel/1  "<Heat Recovered; MBtu/hr>"
  Bus Creator2/1 -> Bus Selector7/1, Out1/1  "CHPData"
  NG_3_5_MVA_Generator/3(Digital Inputs) -> Out2/1
  In2/1 -> CHPThermalModel/5  "CHP_SIM_Cmds"
  NG_3_5_MVA_Generator/10(Gen1 GCB Control) -> GCB Control/1  "Logic_trip"
  CHPThermalModel/4 -> Bus Creator2/5
  CHPThermalModel/5 -> Bus Creator2/6
  Bus Selector7/6 -> Mux1/6  "<Boiler_Nm^3/hr >"
  Bus Selector7/7 -> Mux1/7  "<Boiler lbm/hr CO2 >"
  connections:
  NG_3_5_MVA_Generator/RConn3 -- C/RConn1
  NG_3_5_MVA_Generator/RConn2 -- B/RConn1
  NG_3_5_MVA_Generator/RConn1 -- A/RConn1

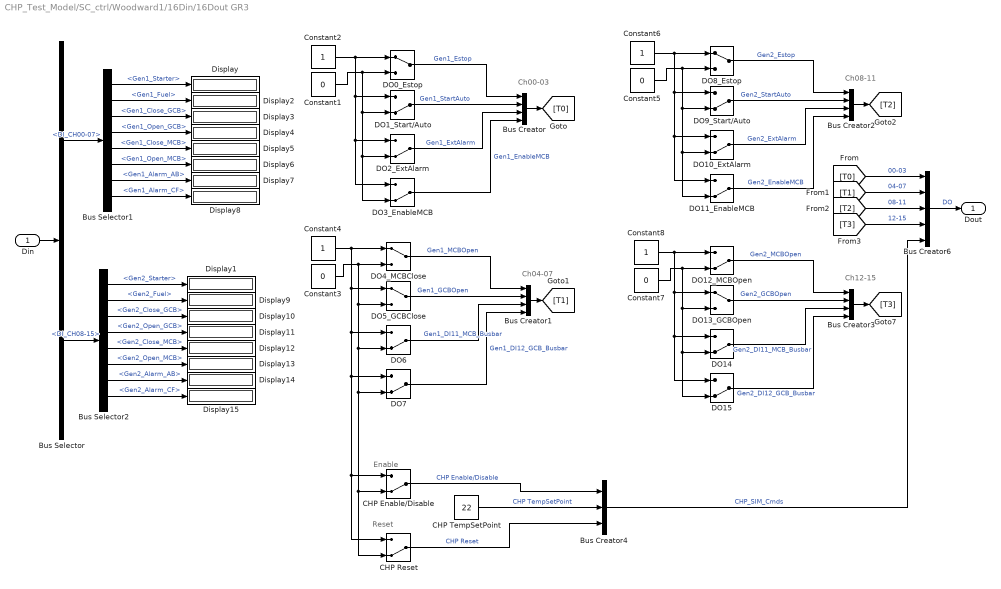
== system CHP_Test_Model/SC_ctrl/Woodward1/16Din/16Dout GR3 ==
  note: Reset
  note: Enable
  note: Ch12-15
  note: Ch08-11
  note: Ch04-07
  note: Ch00-03
  Din : Inport
  Bus Creator{,1..3} (4 alike) : BusCreator
  Bus Creator4 : BusCreator  Inputs=3
  Bus Creator6 : BusCreator  Inputs=5
  Bus Selector : BusSelector  OutputSignals=DIN.DI_CH00-07,DIN.DI_CH08-15
  Bus Selector1 : BusSelector  OutputSignals=Gen1_Starter,Gen1_Fuel,Gen1_Close_GCB,Gen1_Open_GCB,Gen1_Close_MCB,Gen1_Open_MCB,Gen1_Alarm_AB,Gen1_Alarm_CF
  Bus Selector2 : BusSelector  OutputSignals=Gen2_Starter,Gen2_Fuel,Gen2_Close_GCB,Gen2_Open_GCB,Gen2_Close_MCB,Gen2_Open_MCB,Gen2_Alarm_AB,Gen2_Alarm_CF
  CHP Enable/Disable : ManualSwitch  CurrentSetting=0
  CHP Reset : ManualSwitch  CurrentSetting=0
  CHP TempSetPoint : Constant  Value=22
  Constant{1,3,5,7} (4 alike) : Constant  Value=0
  Constant{2,4,6,8} (4 alike) : Constant
  DO0_Estop : ManualSwitch
  DO10_ExtAlarm : ManualSwitch  CurrentSetting=0
  DO11_EnableMCB : ManualSwitch  CurrentSetting=0
  DO12_MCBOpen : ManualSwitch  CurrentSetting=0
  DO13_GCBOpen : ManualSwitch
  DO{6..7,14..15} (4 alike) : ManualSwitch  CurrentSetting=0
  DO1_Start/Auto : ManualSwitch  CurrentSetting=0
  DO2_ExtAlarm : ManualSwitch  CurrentSetting=0
  DO3_EnableMCB : ManualSwitch  CurrentSetting=0
  DO4_MCBClose : ManualSwitch
  DO5_GCBClose : ManualSwitch
  DO8_Estop : ManualSwitch
  DO9_Start/Auto : ManualSwitch  CurrentSetting=0
  Display{,1..15} (16 alike) : Display
  Dout : Outport
  wires:
  Bus Selector1/7 -> Display7/1  "<Gen1_Alarm_AB>"
  Bus Selector1/4 -> Display4/1  "<Gen1_Open_GCB>"
  Bus Selector2/8 -> Display15/1  "<Gen2_Alarm_CF>"
  Bus Selector2/7 -> Display14/1  "<Gen2_Alarm_AB>"
  Bus Selector2/6 -> Display13/1  "<Gen2_Open_MCB>"
  Bus Selector2/5 -> Display12/1  "<Gen2_Close_MCB>"
  Bus Selector2/4 -> Display11/1  "<Gen2_Open_GCB>"
  Bus Selector2/3 -> Display10/1  "<Gen2_Close_GCB>"
  Bus Selector2/2 -> Display9/1  "<Gen2_Fuel>"
  Bus Selector2/1 -> Display1/1  "<Gen2_Starter>"
  Bus Selector/2 -> Bus Selector2/1  "<DI_CH08-15>"
  Bus Selector1/8 -> Display8/1  "<Gen1_Alarm_CF>"
  Bus Selector1/6 -> Display6/1  "<Gen1_Open_MCB>"
  Bus Selector1/5 -> Display5/1  "<Gen1_Close_MCB>"
  Bus Selector1/3 -> Display3/1  "<Gen1_Close_GCB>"
  Bus Selector1/2 -> Display2/1  "<Gen1_Fuel>"
  Bus Selector1/1 -> Display/1  "<Gen1_Starter>"
  Bus Selector/1 -> Bus Selector1/1  "<DI_CH00-07>"
  Din/1 -> Bus Selector/1
  [T3] -> Bus Creator6/4  "12-15"
  [T2] -> Bus Creator6/3  "08-11"
  [T1] -> Bus Creator6/2  "04-07"
  [T0] -> Bus Creator6/1  "00-03"
  Bus Creator2/1 -> [T2]
  Bus Creator3/1 -> [T3]
  Bus Creator1/1 -> [T1]
  Bus Creator/1 -> [T0]
  DO15/1 -> Bus Creator3/4  "Gen2_DI12_GCB_Busbar"
  DO14/1 -> Bus Creator3/3  "Gen2_DI11_MCB_Busbar"
  DO13_GCBOpen/1 -> Bus Creator3/2  "Gen2_GCBOpen"
  DO12_MCBOpen/1 -> Bus Creator3/1  "Gen2_MCBOpen"
  Constant7/1 -> DO12_MCBOpen/2, DO13_GCBOpen/2, DO15/2, DO14/2
  Constant8/1 -> DO12_MCBOpen/1, DO13_GCBOpen/1, DO15/1, DO14/1
  DO11_EnableMCB/1 -> Bus Creator2/4  "Gen2_EnableMCB"
  DO10_ExtAlarm/1 -> Bus Creator2/3  "Gen2_ExtAlarm"
  DO9_Start/Auto/1 -> Bus Creator2/2  "Gen2_StartAuto"
  DO8_Estop/1 -> Bus Creator2/1  "Gen2_Estop"
  Constant5/1 -> DO10_ExtAlarm/2, DO11_EnableMCB/2, DO9_Start/Auto/2, DO8_Estop/2
  Constant6/1 -> DO10_ExtAlarm/1, DO11_EnableMCB/1, DO9_Start/Auto/1, DO8_Estop/1
  DO7/1 -> Bus Creator1/4  "Gen1_DI12_GCB_Busbar"
  DO6/1 -> Bus Creator1/3  "Gen1_DI11_MCB_Busbar"
  DO5_GCBClose/1 -> Bus Creator1/2  "Gen1_GCBOpen"
  DO4_MCBClose/1 -> Bus Creator1/1  "Gen1_MCBOpen"
  Constant3/1 -> DO4_MCBClose/2, DO5_GCBClose/2, DO7/2, CHP Reset/2, CHP Enable/Disable/2, DO6/2
  Constant4/1 -> DO4_MCBClose/1, DO5_GCBClose/1, CHP Reset/1, CHP Enable/Disable/1, DO7/1, DO6/1
  DO3_EnableMCB/1 -> Bus Creator/4  "Gen1_EnableMCB"
  DO2_ExtAlarm/1 -> Bus Creator/3  "Gen1_ExtAlarm"
  DO1_Start/Auto/1 -> Bus Creator/2  "Gen1_StartAuto"
  DO0_Estop/1 -> Bus Creator/1  "Gen1_Estop"
  Constant1/1 -> DO2_ExtAlarm/2, DO3_EnableMCB/2, DO1_Start/Auto/2, DO0_Estop/2
  Constant2/1 -> DO2_ExtAlarm/1, DO3_EnableMCB/1, DO1_Start/Auto/1, DO0_Estop/1
  Bus Creator6/1 -> Dout/1  "DO"
  CHP Enable/Disable/1 -> Bus Creator4/1  "CHP Enable/Disable"
  CHP TempSetPoint/1 -> Bus Creator4/2  "CHP TempSetPoint"
  CHP Reset/1 -> Bus Creator4/3  "CHP Reset"
  Bus Creator4/1 -> Bus Creator6/5  "CHP_SIM_Cmds"

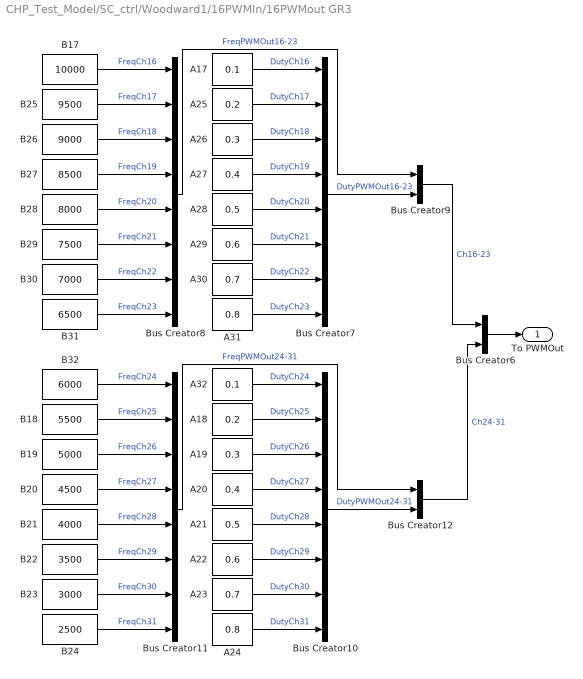
== system CHP_Test_Model/SC_ctrl/Woodward1/16PWMIn/16PWMout GR3 ==
  A17 : Constant  Value=0.1
  A18 : Constant  Value=0.2
  A19 : Constant  Value=0.3
  A20 : Constant  Value=0.4
  A21 : Constant  Value=0.5
  A22 : Constant  Value=0.6
  A23 : Constant  Value=0.7
  A24 : Constant  Value=0.8
  A25 : Constant  Value=0.2
  A26 : Constant  Value=0.3
  A27 : Constant  Value=0.4
  A28 : Constant  Value=0.5
  A29 : Constant  Value=0.6
  A30 : Constant  Value=0.7
  A31 : Constant  Value=0.8
  A32 : Constant  Value=0.1
  B17 : Constant  Value=10000
  B18 : Constant  Value=5500
  B19 : Constant  Value=5000
  B20 : Constant  Value=4500
  B21 : Constant  Value=4000
  B22 : Constant  Value=3500
  B23 : Constant  Value=3000
  B24 : Constant  Value=2500
  B25 : Constant  Value=9500
  B26 : Constant  Value=9000
  B27 : Constant  Value=8500
  B28 : Constant  Value=8000
  B29 : Constant  Value=7500
  B30 : Constant  Value=7000
  B31 : Constant  Value=6500
  B32 : Constant  Value=6000
  Bus Creator{7..8,10..11} (4 alike) : BusCreator  Inputs=8
  Bus Creator12 : BusCreator  Inputs=2
  Bus Creator6 : BusCreator  Inputs=2
  Bus Creator9 : BusCreator  Inputs=2
  To PWMOut : Outport
  wires:
  Bus Creator9/1 -> Bus Creator6/1  "Ch16-23"
  Bus Creator12/1 -> Bus Creator6/2  "Ch24-31"
  Bus Creator11/1 -> Bus Creator12/1  "FreqPWMOut24-31"
  Bus Creator10/1 -> Bus Creator12/2  "DutyPWMOut24-31"
  B24/1 -> Bus Creator11/8  "FreqCh31"
  B23/1 -> Bus Creator11/7  "FreqCh30"
  B22/1 -> Bus Creator11/6  "FreqCh29"
  B21/1 -> Bus Creator11/5  "FreqCh28"
  B20/1 -> Bus Creator11/4  "FreqCh27"
  B19/1 -> Bus Creator11/3  "FreqCh26"
  B18/1 -> Bus Creator11/2  "FreqCh25"
  B32/1 -> Bus Creator11/1  "FreqCh24"
  A24/1 -> Bus Creator10/8  "DutyCh31"
  A23/1 -> Bus Creator10/7  "DutyCh30"
  A22/1 -> Bus Creator10/6  "DutyCh29"
  A21/1 -> Bus Creator10/5  "DutyCh28"
  A20/1 -> Bus Creator10/4  "DutyCh27"
  A19/1 -> Bus Creator10/3  "DutyCh26"
  A18/1 -> Bus Creator10/2  "DutyCh25"
  A32/1 -> Bus Creator10/1  "DutyCh24"
  Bus Creator8/1 -> Bus Creator9/1  "FreqPWMOut16-23"
  Bus Creator7/1 -> Bus Creator9/2  "DutyPWMOut16-23"
  B31/1 -> Bus Creator8/8  "FreqCh23"
  B30/1 -> Bus Creator8/7  "FreqCh22"
  B29/1 -> Bus Creator8/6  "FreqCh21"
  B28/1 -> Bus Creator8/5  "FreqCh20"
  B27/1 -> Bus Creator8/4  "FreqCh19"
  B26/1 -> Bus Creator8/3  "FreqCh18"
  B25/1 -> Bus Creator8/2  "FreqCh17"
  B17/1 -> Bus Creator8/1  "FreqCh16"
  A31/1 -> Bus Creator7/8  "DutyCh23"
  A30/1 -> Bus Creator7/7  "DutyCh22"
  A29/1 -> Bus Creator7/6  "DutyCh21"
  A28/1 -> Bus Creator7/5  "DutyCh20"
  A27/1 -> Bus Creator7/4  "DutyCh19"
  A26/1 -> Bus Creator7/3  "DutyCh18"
  A25/1 -> Bus Creator7/2  "DutyCh17"
  A17/1 -> Bus Creator7/1  "DutyCh16"
  Bus Creator6/1 -> To PWMOut/1

== system CHP_Test_Model/SC_ctrl/Woodward1/16TSDIn/16 TSDOut GR3 ==
  Bus Creator1 : BusCreator  Inputs=3
  Din/Dout ch16-23 : Subsystem
  Din/Dout ch24-31 : Subsystem
  Dout state ctrl : Subsystem
  TSDout : Outport
  wires:
  Bus Creator1/1 -> TSDout/1
  Dout state ctrl/1(Event State OUT) -> Bus Creator1/3  "states"
  Din/Dout ch16-23/1(Out1) -> Bus Creator1/1  "times CH16-23"
  Din/Dout ch24-31/1(Out1) -> Bus Creator1/2  "times CH24-31"

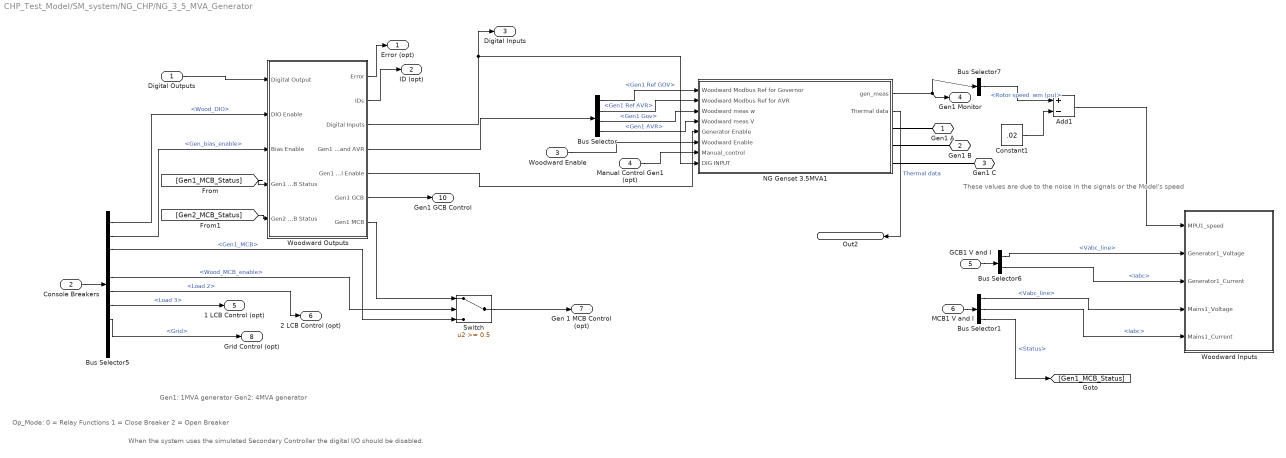
== system CHP_Test_Model/SM_system/NG_CHP/NG_3_5_MVA_Generator ==
  note: When the system uses the simulated
      | Secondary Controller the digital I/O
      | should be disabled.
  note: Gen1: 1MVA generator
      | Gen2: 4MVA generator
  note: These values are due to
      | the noise in the signals
      | or the Model's speed
  note: Op_Mode:
      | 0 = Relay Functions
      | 1 = Close Breaker
      | 2 = Open Breaker
  Digital Outputs : Inport
  Console Breakers : Inport  Port=2
  Woodward Enable : Inport  Port=3
  Manual Control Gen1 (opt) : Inport  Port=4
  GCB1 V and I : Inport  Port=5
  MCB1 V and I : Inport  Port=6
  Add1 : Sum  Inputs=+-
  Bus Selector : BusSelector  OutputSignals=Gen1 Ref GOV,Gen1 Ref AVR,Gen1 Gov,Gen1 AVR
  Bus Selector1 : BusSelector  OutputSignals=Vabc_line,Iabc,Status
  Bus Selector5 : BusSelector  OutputSignals=Wood_DIO,Gen_bias_enable,Gen1_MCB,Gen2_MCB,Wood_MCB_enable,Load 2,Load 3,Grid,Gen2_enable,Load 1
  Bus Selector6 : BusSelector  OutputSignals=Vabc_line,Iabc
  Bus Selector7 : BusSelector  OutputSignals="w.w.Rotor speed  wm (pu)"
  Constant1 : Constant  Value=.02
  NG Genset 3.5MVA1 : Subsystem  mask(Gen-Set with simulated control modes){control_mode=1}
      mask prompts: control_mode "Control Mode [0 => Sim. 1 => Wood.]"
      mask help:
      | This Gen-Set block allows the user to indicate the control mode of the generator. The available control modes are: (1) PQ, (2) PV, and (3) VF.
      | The input values to the block will be applied according to the selected control mode.
      | For example, if PQ mode is selected, the controller will only work based on P_ref and Q_ref ignoring values of other inputs to the block.
  Switch : Switch  Threshold=0.5
  Woodward Inputs : Subsystem
  Woodward Outputs : Subsystem
  Gen1 A : PMIOPort  Port=1  Side=Right
  Gen1 B : PMIOPort  Port=2  Side=Right
  Gen1 C : PMIOPort  Port=3  Side=Right
  Error (opt) : Outport
  ID (opt) : Outport  Port=2
  Digital Inputs : Outport  Port=3
  Gen1 Monitor : Outport  Port=4
  1 LCB Control (opt) : Outport  Port=5
  2 LCB Control (opt) : Outport  Port=6
  Gen 1 MCB Control (opt) : Outport  Port=7
  Grid Control (opt) : Outport  Port=8
  Out2 : Outport  Port=9
  Gen1 GCB Control : Outport  Port=10
  wires:
  Woodward Outputs/3(Digital Inputs) -> Digital Inputs/1, NG Genset 3.5MVA1/8(DIG INPUT)
  Add1/1 -> Woodward Inputs/1(MPU1_speed)
  NG Genset 3.5MVA1/2(Thermal data) -> Out2/1  "Thermal data"
  Constant1/1 -> Add1/2
  Bus Selector5/8 -> Grid Control (opt)/1  "<Grid>"
  Bus Selector5/3 -> Switch/3  "<Gen1_MCB>"
  Bus Selector5/6 -> 2 LCB Control (opt)/1  "<Load 2>"
  [Gen2_MCB_Status] -> Woodward Outputs/5(Gen2 MCB Status)
  [Gen1_MCB_Status] -> Woodward Outputs/4(Gen1 MCB Status)
  Bus Selector/4 -> NG Genset 3.5MVA1/4(Woodward meas V)  "<Gen1 AVR>"
  Bus Selector/3 -> NG Genset 3.5MVA1/3(Woodward meas w)  "<Gen1 Gov>"
  Bus Selector/2 -> NG Genset 3.5MVA1/2(Woodward Modbus Ref for AVR)  "<Gen1 Ref AVR>"
  Bus Selector/1 -> NG Genset 3.5MVA1/1(Woodward Modbus Ref for Governor)  "<Gen1 Ref GOV>"
  Woodward Outputs/4(Gen1 Gov and AVR) -> Bus Selector/1
  Bus Selector1/2 -> Woodward Inputs/5(Mains1_Current)  "<Iabc>"
  Bus Selector1/1 -> Woodward Inputs/4(Mains1_Voltage)  "<Vabc_line>"
  MCB1 V and I/1 -> Bus Selector1/1
  Switch/1 -> Gen 1 MCB Control (opt)/1
  Bus Selector5/7 -> 1 LCB Control (opt)/1  "<Load 3>"
  Console Breakers/1 -> Bus Selector5/1
  Woodward Outputs/6(Gen1 GCB) -> Gen1 GCB Control/1
  GCB1 V and I/1 -> Bus Selector6/1
  Digital Outputs/1 -> Woodward Outputs/1(Digital Output)
  Woodward Outputs/7(Gen1 MCB) -> Switch/1
  Bus Selector5/5 -> Switch/2  "<Wood_MCB_enable>"
  Woodward Outputs/5(Gen1 Fuel Enable) -> NG Genset 3.5MVA1/5(Generator Enable)
  Woodward Enable/1 -> NG Genset 3.5MVA1/6(Woodward Enable)
  Woodward Outputs/2(IDs) -> ID (opt)/1
  Woodward Outputs/1(Error) -> Error (opt)/1
  Bus Selector7/1 -> Add1/1  "<Rotor speed  wm (pu)>"
  Bus Selector5/2 -> Woodward Outputs/3(Bias Enable)  "<Gen_bias_enable>"
  Manual Control Gen1 (opt)/1 -> NG Genset 3.5MVA1/7(Manual_control)
  Bus Selector5/1 -> Woodward Outputs/2(DIO Enable)  "<Wood_DIO>"
  Bus Selector6/2 -> Woodward Inputs/3(Generator1_Current)  "<Iabc>"
  Bus Selector6/1 -> Woodward Inputs/2(Generator1_Voltage)  "<Vabc_line>"
  NG Genset 3.5MVA1/1(gen_meas) -> Gen1 Monitor/1, Bus Selector7/1
  Bus Selector1/3 -> [Gen1_MCB_Status]  "<Status>"
  connections:
  NG Genset 3.5MVA1/RConn3 -- Gen1 C/RConn1
  NG Genset 3.5MVA1/RConn2 -- Gen1 B/RConn1
  NG Genset 3.5MVA1/RConn1 -- Gen1 A/RConn1

== system CHP_Test_Model/SC_ctrl/Woodward1/16TSDIn/16 TSDOut GR3/Din/Dout ch16-23 ==
  Bus Creator3 : BusCreator  Inputs=8
  times17 : Constant  Value=[0.05 0.15 0.25 0.35]
  times18 : Constant  Value=[0.1 0.2 0.3 0.4]
  times19 : Constant  Value=[0.15 0.25 0.35 0.45]
  times20 : Constant  Value=[0.2 0.3 0.4 0.5]
  times21 : Constant  Value=[0.25 0.35 0.45 0.55]
  times22 : Constant  Value=[0.3 0.4 0.5 0.6]
  times23 : Constant  Value=[0.3 0.4 0.5 0.6]
  times24 : Constant  Value=[0 0.1 0.2 0.3]
  Out1 : Outport
  wires:
  times24/1 -> Bus Creator3/1  "times17"
  times17/1 -> Bus Creator3/2  "times18"
  times18/1 -> Bus Creator3/3  "times19"
  times19/1 -> Bus Creator3/4  "times20"
  times20/1 -> Bus Creator3/5  "times21"
  times21/1 -> Bus Creator3/6  "times22"
  times22/1 -> Bus Creator3/7  "times23"
  times23/1 -> Bus Creator3/8  "times24"
  Bus Creator3/1 -> Out1/1

== system CHP_Test_Model/SC_ctrl/Woodward1/16TSDIn/16 TSDOut GR3/Din/Dout ch24-31 ==
  Bus Creator4 : BusCreator  Inputs=8
  times25 : Constant  Value=[0.05 0.15 0.25 0.35]
  times26 : Constant  Value=[0.1 0.2 0.3 0.4]
  times27 : Constant  Value=[0.15 0.25 0.35 0.45]
  times28 : Constant  Value=[0.2 0.3 0.4 0.5]
  times29 : Constant  Value=[0.25 0.35 0.45 0.55]
  times30 : Constant  Value=[0.3 0.4 0.5 0.6]
  times31 : Constant  Value=[0.3 0.4 0.5 0.6]
  times32 : Constant  Value=[0 0.1 0.2 0.3]
  Out1 : Outport
  wires:
  times32/1 -> Bus Creator4/1  "times25"
  times25/1 -> Bus Creator4/2  "times26"
  times26/1 -> Bus Creator4/3  "times27"
  times27/1 -> Bus Creator4/4  "times28"
  times28/1 -> Bus Creator4/5  "times29"
  times29/1 -> Bus Creator4/6  "times30"
  times30/1 -> Bus Creator4/7  "times31"
  times31/1 -> Bus Creator4/8  "times32"
  Bus Creator4/1 -> Out1/1

== system CHP_Test_Model/SC_ctrl/Woodward1/16TSDIn/16 TSDOut GR3/Dout state ctrl ==
  Bus Creator : BusCreator  Inputs=2
  Dout_CH16_CH23 : Subsystem
  Dout_CH24_CH31 : Subsystem
  Event State OUT : Outport
  wires:
  Bus Creator/1 -> Event State OUT/1
  Dout_CH16_CH23/1(Dout_CH8_CH15) -> Bus Creator/1  "CH16-23"
  Dout_CH24_CH31/1(Dout_CH8_CH15) -> Bus Creator/2  "CH24-31"
